simulink library "commchan"  (Simulink 5.0)
values from neighbouring files (symbols this model uses):
  b = []    [commblkvfdly.m]    (also in eyesampl.m = findobj(a, 'Name', get_param(gcbh,'Name')))
  params = []    [commblkeyescatdisc.m]
undefined symbols (not defined in the file or in its folder): j
libraries: dspsrcs2 x2, commsource x2, dspmlti2 x2, dsparch2 x1, dspelem2 x1, dspmtrx2 x1, commchan x1
settings Model: RequirementInfo=9  Creator=tdelve  LastModifiedBy=mmclerno

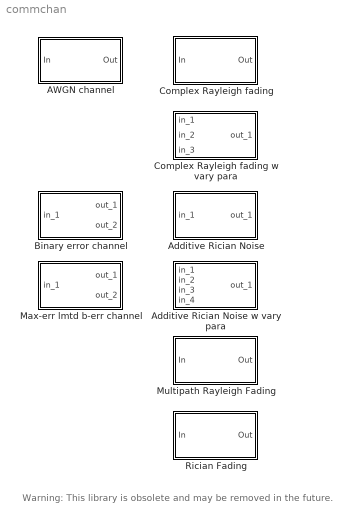
== system commchan ==
  note: Warning:  This library is obsolete and may
      | be removed in the future.
  AWGN channel : Subsystem  mask(AWGN Channel){seed=123456, noiseMode=Signal to noise ratio  (Es/No), EsNodB=10, SNRdB=10, Ps=1, Tsym=1, variance=1, FrameBased=off, nChans=1}
      mask prompts: seed "Initial seed:"; noiseMode "Mode:"; EsNodB "Es/No (dB):"; SNRdB "SNR (dB):"; Ps "Input signal power (Watts):"; Tsym "Symbol period (sec):"; FrameBased "Frame-based inputs"; nChans "Number of channels:"
      mask help:
      | Add white Gaussian noise to the input signal. The input and output signals can be real or complex. This block supports multi channel input and output signals as well as frame-based processing.
      |
      | When using either of the variance modes with complex inputs, the variance values are equally divided among the real and imaginary components of the input signal.
      mask init:
      | [mode,s]=commblkawgnchan(gcb,'init');
      mask StyleString: edit,popup(Signal to noise ratio  (Es/No)|Signal to noise ratio  (SNR)|Variance from mask|Variance from port),edit,edit,edit,edit,edit,checkbox,edit
      mask CallbackString: |commblkawgnchan(gcb,'Mode');||||||commblkawgnchan(gcb,'FrameBased');|
      mask Display:
      | plot(-10,-10,110, 110,[05 15 10 10 05 10 18 14 13 7.5 13 41 44 47 50 53 57
      | 59 100-[13 7.5 13 14 18 10 5 10 10 15 5]],[70 70 70 85 92 85 79 82 90 88.5
      | 90 90 87 93 87 93 87 90 90 88.5 90 82 79 85 92 85 70 70 70]);
      | disp('AWGN');
      | port_label('input',s.i1,s.i1s);
      | port_label('input',s.i2,s.i2s);
      | port_label('output',s.o1,s.o1s);
  Additive Rician Noise : Subsystem  mask(Rician noise channel, fixed parameter){m1=.1, m2=.3, d=.1, s=1234}
      mask prompts: m1 "In-phase mean:"; m2 "Quadrature mean:"; d "Variance:"; s "Seed:"
      mask help: Additive Rician noise channel for baseband signal simulation. Input and output signals are complex.
      mask init:
      | rand('state',s(1));
      | SeedVec = floor(1e5*rand(2,1));
      mask Help: This block adds Rician noise to the input signal. The input and output of this block are complex signals. Rician noise is composed of two independant Gaussian noise elements. The two Gaussian components have the same variance. Their mean values are in-phase mean and quadrature mean respectively.
      mask Display:
      | plot(0,0,100,100,[05 15 10 10 05 10 18 14 13 7.5 13 41 44 47 50 53 57 59 100-[13 7.5 13 14 18 10 5 10 10 15 5]],[70 70 70 85 92 85 79 82 90 88.5 90 90 87 93 87 93 87 90 90 88.5 90 82 79 85 92 85 70 70 70]);
      | disp('Complex\nRician Noise')
  Additive Rician Noise w vary para : Subsystem  mask(Rician noise channel, vary parameter){s=[13579,  24680]}
      mask prompts: s "Seeds:"
      mask help: Add Rician noise to complex signal (1st port) with the varying in-phase mean (2nd port), quadrature mean (3rd port), and variance (4th port).
      mask init:
      | rand('state',s(1));
      | SeedVec = floor(1e5*rand(2,1));
      mask Help: This block adds Rician noise to the transmitted signal. The 1st port input and output of this block are complex data. The Rician noise is composed of two independant Gaussian noise elements. The mean value of the two Gaussian components are input from 2nd and 3rd inports respectively. Their variance are the same which is input from the 4th inport.
      mask Display:
      | plot(0,0,100,100,[05 15 10 10 05 10 18 14 13 7.5 13 41 44 47 50 53 57 59 100-[13 7.5 13 14 18 10 5 10 10 15 5]],[70 70 70 85 92 85 79 82 90 88.5 90 90 87 93 87 93 87 90 90 88.5 90 82 79 85 92 85 70 70 70]);
      | disp('Complex\nRician Noise')
  Binary error channel : Subsystem  mask(Binary Error Channel){P=0.05, M=15, s=12345, Ts=1}
      mask prompts: P "Error probability:"; M "Input vector length:"; s "Seed"; Ts "Sample time (s):"
      mask help: Add binary errors to the input signal. The error probability can be a scalar or a vector with the same length as the input vector length.
      mask init:
      | if length(P)~=M,P=ones(1,M)*P(1);end;
      | seed = s(1)+cumsum(ones(1,M));
      mask Help: This block adds binary errors to transmitted binary signals. The error probability is given in the parameter setting. The first output port outputs the transmitting signal (after adding noise). The second port outputs the errors signal added to the transmitting signal.
      mask Display:
      | plot(0,0,100,100,[05 15 10 10 05 10 18 14 13 7.5 13 41 44 47 50 53 57 59 100-[13 7.5 13 14 18 10 5 10 10 15 5]],[70 70 70 85 92 85 79 82 90 88.5 90 90 87 93 87 93 87 90 90 88.5 90 82 79 85 92 85 70 70 70]);
      | disp('B-error')
  Complex Rayleigh fading : Subsystem  mask(Rayleigh fading channel, fixed parameter){a=1, Ph=0}
      mask prompts: a "Rayleigh fading envelope:"; Ph "Phase shift of the channel (rad):"
      mask help: Rayleigh fading channel with fixed fading envelope and phase shift.
      mask Help: This block applies the fading and phase shifting to the transmitting signal. In general, the fading envelope should be no larger than one. The input and the output of this block are both complex signals.
      mask Display:
      | plot(0,0,100,100,[05 15 10 10 05 10 18 14 13 7.5 13 41 44 47 50 53 57 59 100-[13 7.5 13 14 18 10 5 10 10 15 5]],[70 70 70 85 92 85 79 82 90 88.5 90 90 87 93 87 93 87 90 90 88.5 90 82 79 85 92 85 70 70 70]);
      | disp('Complex\nRayl Fading')
  Complex Rayleigh fading w vary para : Subsystem
      mask Type: Rayleigh fading channel, vary parameter
      mask Description: The fading envelope and the phase shift of the channel changes with the 2nd and 3rd input port values.
      mask Help: This block applies Rayleigh fading to the transmitting signals. The fading envelope and the phase of the channel are provided in the 2nd and the 3rd input port. The 1st input port and the output of this block are complex signals.
      mask Display:
      | plot(0,0,100,100,[05 15 10 10 05 10 18 14 13 7.5 13 41 44 47 50 53 57 59 100-[13 7.5 13 14 18 10 5 10 10 15 5]],[70 70 70 85 92 85 79 82 90 88.5 90 90 87 93 87 93 87 90 90 88.5 90 82 79 85 92 85 70 70 70]);
      | disp('Complex\nRayl Fading')
  Max-err lmtd b-err channel : Subsystem  mask(Limited binary error channel){leng=7, prob=1/2, seed=12345, Ts=}
      mask prompts: leng "Vector length(can't be changed during simulation):"; prob "Probability of one err, two errs, three errs...:"; Ts "Sample time (s):"
      mask help: Add binary errors with specified error number probability.
      mask Help: This block adds binary errors to the input signal. The maximum number of errors added to the signal is the same as the length of the vector probability. The value of ith element of the probability is the probability of i number of errors in the vector. The 1st outport is the signal with added noise. The 2nd outport is the added noise.
      mask Display:
      | plot(0,0,100,100,[05 15 10 10 05 10 18 14 13 7.5 13 41 44 47 50 53 57 59 100-[13 7.5 13 14 18 10 5 10 10 15 5]],[70 70 70 85 92 85 79 82 90 88.5 90 90 87 93 87 93 87 90 90 88.5 90 82 79 85 92 85 70 70 70]);
      | disp('Lmtd b-err')
  Multipath Rayleigh Fading : Subsystem  mask(Multipath Rayleigh Fading){Fd=40, simTs=1e-6, delayVec=[0 2e-6], gainVecdB=[0 -3], normGain=on, Seed=1234}
      mask prompts: Fd "Doppler frequency (Hz):"; simTs "Sample time (sec):"; delayVec "Delay vector (sec):"; gainVecdB "Gain vector (dB):"; normGain "Normalize gain vector to 0 dB overall gain"; Seed "Initial seed:"
      mask help:
      | Multipath Rayleigh fading channel for complex baseband signals.
      |
      | Multiplies the input signal with samples of a Rayleigh distributed complex random process. The spectrum of the Rayleigh process is given by the Jakes PSD, where the Doppler frequency parameter determines the maximum Doppler frequency.
      |
      | The number of paths equals the length of either the 'Delay vector' or 'Gain vector' parameters.
      mask init:
      | commblkrayleighchan(gcb);
      mask Help: web(commbhelp);
      mask Display:
      | plot(0,0,100,100,[05 15 10 10 05 10 18 14 13 7.5 13 41 44 47 50 53 57 59 100-[13 7.5 13 14 18 10 5 10 10 15 5]],[70 70 70 85 92 85 79 82 90 88.5 90 90 87 93 87 93 87 90 90 88.5 90 82 79 85 92 85 70 70 70]);
      | disp('Multipath\nRayleigh Fading')
  Rician Fading : Subsystem  mask(Rician Fading){K=1, Fd=40, simTs=1e-6, delayVec=0, gainVecdB=0, Seed=1234}
      mask prompts: K "K-factor:"; Fd "Doppler frequency (Hz):"; simTs "Sample time (sec):"; delayVec "Delay (sec):"; gainVecdB "Gain (dB):"; Seed "Initial seed:"
      mask help:
      | Rician fading channel for complex baseband signals.
      |
      | Multiplies the input signal with samples of a Rician distributed complex random process. The K-factor parameter specifies the linear ratio of power in the direct path to the diffuse power.  The spectrum of the Rician process is given by the Jakes PSD, where the Doppler frequency parameter determines the maximum Doppler frequency.
      mask init:
      | commblkricianchan(gcb);
      mask Help: web(commbhelp);
      mask Display:
      | plot(0,0,100,100,[05 15 10 10 05 10 18 14 13 7.5 13 41 44 47 50 53 57 59 100-[13 7.5 13 14 18 10 5 10 10 15 5]],[70 70 70 85 92 85 79 82 90 88.5 90 90 87 93 87 93 87 90 90 88.5 90 82 79 85 92 85 70 70 70]);
      | disp('Rician\nFading')

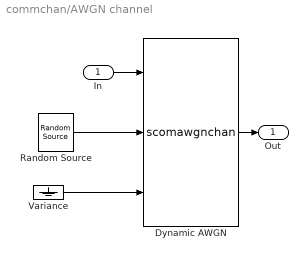
== system commchan/AWGN channel ==
  In : Inport
  Dynamic AWGN : S-Function  FunctionName=scomawgnchan  Parameters=noiseMode,EsNodB,SNRdB,Ps,Tsym,variance,FrameBased,nChans
  Random Source : dspsrcs2/Random Source  SrcType=Gaussian  Min=0  Max=1  Mean=0  Var=1  Seed=seed  SampMode=Discrete  Inherit=on  SampTime=1  SampFrame=1  OutComplex=Real
  Variance : Ground
  Out : Outport
  wires:
  Random Source/1 -> Dynamic AWGN/2
  In/1 -> Dynamic AWGN/1
  Dynamic AWGN/1 -> Out/1
  Variance/1 -> Dynamic AWGN/3

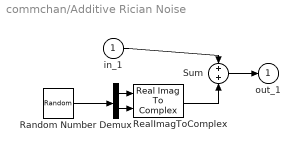
== system commchan/Additive Rician Noise ==
  in_1 : Inport
  Demux : Demux  Outputs=2
  Random Number : RandomNumber  Mean=[m1 m2]  Variance=[d d]  Seed=SeedVec
  RealImagToComplex : RealImagToComplex
  Sum : Sum  SaturateOnIntegerOverflow=on  InputSameDT=on
  out_1 : Outport  InitialOutput=0
  wires:
  Sum/1 -> out_1/1
  in_1/1 -> Sum/1
  RealImagToComplex/1 -> Sum/2
  Demux/1 -> RealImagToComplex/1
  Demux/2 -> RealImagToComplex/2
  Random Number/1 -> Demux/1

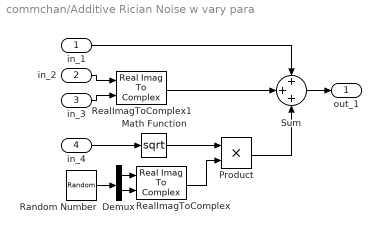
== system commchan/Additive Rician Noise w vary para ==
  in_1 : Inport
  in_2 : Inport  Port=2
  in_3 : Inport  Port=3
  in_4 : Inport  Port=4
  Demux : Demux  Outputs=2
  Math Function : Math  Operator=sqrt
  Product : Product  SaturateOnIntegerOverflow=on  InputSameDT=on
  Random Number : RandomNumber  Seed=SeedVec
  RealImagToComplex : RealImagToComplex
  RealImagToComplex1 : RealImagToComplex
  Sum : Sum  Inputs=+++  SaturateOnIntegerOverflow=on  InputSameDT=on
  out_1 : Outport  InitialOutput=0
  wires:
  in_2/1 -> RealImagToComplex1/1
  in_3/1 -> RealImagToComplex1/2
  RealImagToComplex/1 -> Product/2
  Product/1 -> Sum/3
  RealImagToComplex1/1 -> Sum/2
  in_1/1 -> Sum/1
  Sum/1 -> out_1/1
  Demux/1 -> RealImagToComplex/1
  Demux/2 -> RealImagToComplex/2
  Random Number/1 -> Demux/1
  in_4/1 -> Math Function/1
  Math Function/1 -> Product/1

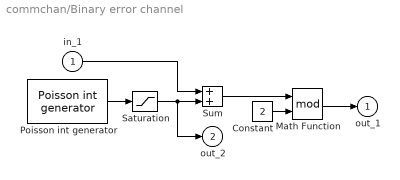
== system commchan/Binary error channel ==
  in_1 : Inport
  Constant : Constant  Value=2
  Math Function : Math  Operator=mod
  Poisson int generator : commsource/Poisson int generator  lambda=P  seed=seed  Ts=Ts
  Saturation : Saturate  UpperLimit=1  LowerLimit=0
  Sum : Sum  SaturateOnIntegerOverflow=on  InputSameDT=on
  out_1 : Outport  InitialOutput=0
  out_2 : Outport  Port=2  InitialOutput=0
  wires:
  Saturation/1 -> Sum/2, out_2/1
  Poisson int generator/1 -> Saturation/1
  in_1/1 -> Sum/1
  Sum/1 -> Math Function/1
  Constant/1 -> Math Function/2
  Math Function/1 -> out_1/1

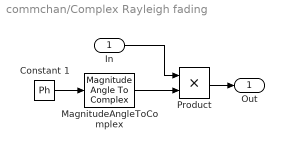
== system commchan/Complex Rayleigh fading ==
  In : Inport
  Constant 1 : Constant  Value=Ph
  MagnitudeAngleToComplex : MagnitudeAngleToComplex  Input=Angle  ConstantPart=a
  Product : Product  SaturateOnIntegerOverflow=on  InputSameDT=on
  Out : Outport  InitialOutput=0
  wires:
  Constant 1/1 -> MagnitudeAngleToComplex/1
  MagnitudeAngleToComplex/1 -> Product/2
  In/1 -> Product/1
  Product/1 -> Out/1

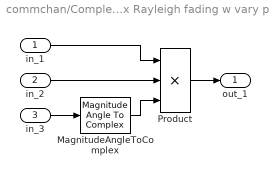
== system commchan/Complex Rayleigh fading w vary para ==
  in_1 : Inport
  in_2 : Inport  Port=2
  in_3 : Inport  Port=3
  MagnitudeAngleToComplex : MagnitudeAngleToComplex  Input=Angle  ConstantPart=1
  Product : Product  Inputs=3  SaturateOnIntegerOverflow=on  InputSameDT=on
  out_1 : Outport  InitialOutput=0
  wires:
  Product/1 -> out_1/1
  in_2/1 -> Product/2
  in_1/1 -> Product/1
  MagnitudeAngleToComplex/1 -> Product/3
  in_3/1 -> MagnitudeAngleToComplex/1

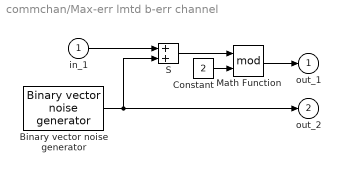
== system commchan/Max-err lmtd b-err channel ==
  in_1 : Inport
  Binary vector noise generator : commsource/Binary vector noise generator  n=leng  prob=prob  seed=seed  Ts=Ts
  Constant : Constant  Value=2
  Math Function : Math  Operator=mod
  S : Sum  SaturateOnIntegerOverflow=on  InputSameDT=on
  out_1 : Outport  InitialOutput=0
  out_2 : Outport  Port=2  InitialOutput=0
  wires:
  S/1 -> Math Function/1
  in_1/1 -> S/1
  Binary vector noise generator/1 -> S/2, out_2/1
  Constant/1 -> Math Function/2
  Math Function/1 -> out_1/1

== system commchan/Multipath Rayleigh Fading ==
  In : Inport
  Multipath Fading Channel : Subsystem  mask(Multipath Fading){Fd=Fd, LOSFd=0, K=0, simTs=simTs, delayVec=delayVec, gainVecdB=gainVecdB, normGain=on, Seed=Seed}
      mask prompts: Fd "Doppler frequency (Hz):"; LOSFd "Line-of-sight Doppler frequency (Hz):"; K "K-factor:"; simTs "Sample time (sec):"; delayVec "Delay vector (sec):"; gainVecdB "Gain vector (dB):"; normGain "Normalize gain vector to 0 dB overall gain"; Seed "Initial seed:"
      mask help:
      | Multipath fading channel for complex baseband signals.
      |
      | Multiplies the input signal with samples of a complex random process. The spectrum of the random process is given by the Jakes PSD, where the Doppler frequency parameter determines the maximum Doppler frequency. The K-factor parameter specifies the linear ratio of power in the direct path to the diffuse power.
      |
      | The number of paths equals the length of either the 'Delay vector' or 'Gain vector' parameters.
      mask init:
      | [ecode,emsg,params] = commblkfadingchan(gcb,Fd,LOSFd,K,simTs,delayVec,gainVecdB,normGain,Seed);
      | if(ecode==1)
      |     error(emsg);
      | elseif(ecode==2)
      |     warning(emsg);
      | end;
      mask Display:
      | plot(0,0,100,100,[05 15 10 10 05 10 18 14 13 7.5 13 41 44 47 50 53 57 59 100-[13 7.5 13 14 18 10 5 10 10 15 5]],[70 70 70 85 92 85 79 82 90 88.5 90 90 87 93 87 93 87 90 90 88.5 90 82 79 85 92 85 70 70 70]);
      | disp('Multipath\nFading')
  Out : Outport
  wires:
  In/1 -> Multipath Fading Channel/1(In)
  Multipath Fading Channel/1(Out) -> Out/1

== system commchan/Rician Fading ==
  In : Inport
  Multipath Fading Channel : commchan/Multipath Rayleigh Fading/Multipath Fading Channel  Fd=Fd  LOSFd=0  K=K  simTs=simTs  delayVec=delayVec  gainVecdB=gainVecdB  normGain=off  Seed=Seed
  Out : Outport
  wires:
  In/1 -> Multipath Fading Channel/1
  Multipath Fading Channel/1 -> Out/1

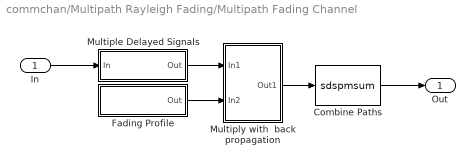
== system commchan/Multipath Rayleigh Fading/Multipath Fading Channel ==
  In : Inport
  Combine Paths : S-Function  FunctionName=sdspmsum  Parameters=Cols,Dim  mask(Matrix Sum){Dim=Rows, Cols=params.nPaths}
      mask prompts: Dim "Sum along:"; Cols "Number of columns in input:"
      mask help: Sum of matrix elements along the row or column dimension.
      mask init:
      | if (Dim==1), str='Row\nSum';
      | else str='Column\nSum';
      | end
      mask Help: web(dspbhelp);
      mask StyleString: popup(Rows|Columns),edit
      mask Display: disp(str);
  Fading Profile : Subsystem
      mask Display: disp('Fading\nProfile')
  Multiple Delayed Signals : Subsystem  mask(Multiple Delayed Signals){delayVector=params.sampleDelayVec, Ts=simTs}
      mask prompts: delayVector "Path delay vector:"; Ts "Sample time (sec):"
      mask init:
      | nPaths = length(delayVector);
      | maxDelay = ceil(max(delayVector))+1;
      mask Display: disp('Multiple\ndelayed signals');
  Multiply with  back propagation : Subsystem  mask(Multiply with back propagation){propTarget=Input 2, Ts=simTs, numChan=params.nPaths}
      mask prompts: propTarget "Propagation target:"; Ts "Sample time:"; numChan "Number of channels:"
      mask help:
      | Perform multiplication of the two input signals.
      |
      | The width and complexity of the output and the port not targeted for propagation must be identical. The width and complexity of the port targeted for propagation is set to that of the other input.
      |
      | The block sample time is the product of the number of samples per frame and the sample time parameter.
      mask StyleString: popup(Input 1|Input 2),edit,edit
      mask Display: disp('Multiply\nwith prop');
  Out : Outport
  wires:
  Multiple Delayed Signals/1(Out) -> Multiply with  back propagation/1(In1)
  Fading Profile/1(Out) -> Multiply with  back propagation/2(In2)
  In/1 -> Multiple Delayed Signals/1(In)
  Multiply with  back propagation/1(Out1) -> Combine Paths/1
  Combine Paths/1 -> Out/1

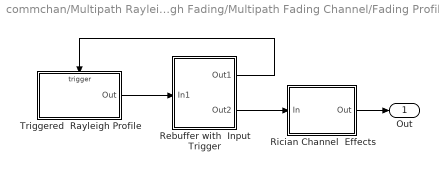
== system commchan/Multipath Rayleigh Fading/Multipath Fading Channel/Fading Profile ==
  Rebuffer with  Input Trigger : Subsystem  mask(Rebuffer with Input Trigger){startSample=params.startDelay, numChan=params.nPaths, inputWidthMode=Based on output width, inputWidth=params.intFactor, inputWidthMin=params.intFactor, inputWidthStep=params.intFactor, inputWidthMax=params.maxPathWidth}
      mask prompts: startSample "Start delay:"; numChan "Number of channels:"; inputWidthMode "Input width mode:"; inputWidth "Input width (per channel):"; inputWidthMin "Minimum input width (per channel):"; inputWidthStep "Input width step size (per channel):"; inputWidthMax "Maximum input width (per channel):"
      mask help: This block inherits the input and output port widths and complexity and the output sample time. The input must be from a function call subsystem. The block generates a function call trigger on port 1 when ever data is required. and outputs the buffered input data on port 2.
      mask init:
      | s = commblktriggeredbuffer(gcb,'init',{});
      mask StyleString: edit,edit,popup(Inherit|Specify|Based on output width),edit,edit,edit,edit
      mask CallbackString: ||commblktriggeredbuffer(gcb,'InputWidthMode');||||
      mask Display:
      | disp('Rebuffer\nwith trigger');
      | port_label('input',s.i1,s.i1s);
      | port_label('output',s.o1,s.o1s);
      | port_label('output',s.o2,s.o2s);
  Rician Channel  Effects : Subsystem  mask(Ricean Channel Effects){Doppler=params.LOSFd, K=params.K, opPower=params.gainVecLin, Ts=simTs, numChan=params.nPaths}
      mask prompts: Doppler "Line-of-sight Doppler frequency (Hz):"; K "K-factor"; opPower "Required output power (Watts):"; Ts "Sample time (s):"; numChan "Number of channels:"
      mask help: Add a complex phasor to the unity variance complex input to produce Rician channel effects. The Doppler frequency parameter determines frequency of the complex phasor.
      mask Display: disp('Rician\nChannel')
  Triggered  Rayleigh Profile : Subsystem  TreatAsAtomicUnit=on
  Out : Outport
  wires:
  Rebuffer with  Input Trigger/1(Out1) -> Triggered  Rayleigh Profile/Trigger
  Triggered  Rayleigh Profile/1(Out) -> Rebuffer with  Input Trigger/1(In1)
  Rebuffer with  Input Trigger/2(Out2) -> Rician Channel  Effects/1(In)
  Rician Channel  Effects/1(Out) -> Out/1

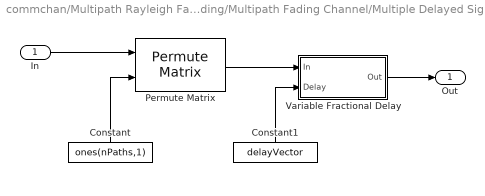
== system commchan/Multipath Rayleigh Fading/Multipath Fading Channel/Multiple Delayed Signals ==
  In : Inport
  Constant : Constant  Orientation=up  Value=ones(nPaths,1)
  Constant1 : Constant  Orientation=up  Value=delayVector
  Permute Matrix : dspmtrx2/Permute Matrix  mode=Columns  errmode=Clip Index  cols=1
  Variable Fractional Delay : Subsystem  mask(Variable Fractional Delay){mode=FIR Interpolation, dmax=maxDelay, L=6, R=10, alpha=1, ic=0, frame=on, numChans=nPaths, delayMode=on}
      mask prompts: dmax "Maximum delay in samples:"; L "Interpolation filter half-length:"; R "Interpolation points per input sample:"; alpha "Normalized input bandwidth (0 to 1):"; ic "Initial Conditions:"; frame "Frame-Based Inputs"; numChans "Number of Channels:"; delayMode "Delay input is "delay per channel""
      mask help: Delay discrete-time input by a time-varying fractional number of sample periods, as specified by the "delay" input. The delay may be applied on an element-by-element basis or channel-by-channel. Delay must be a real vector signal with one delay value per frame element or one delay value per channel when in channel-by-channel mode. The FIR filter is designed using "intfilt" from the Signal Processing Toolbox.
      mask init:
      | [b,str] = commblkvfdly(mode,R,L,alpha);
      | if strcmp(frame,'off'), numChans=-1; end
      mask StyleString: popup(Linear Interpolation|FIR Interpolation),edit,edit,edit,edit,edit,checkbox,edit,checkbox
      mask CallbackString: commblkvfdly||||||commblkvfdly||
      mask Display:
      | text(0.5,0.4,'z','horiz','right')
      | text(0.5,0.6,'-f','horiz','left')
  Out : Outport
  wires:
  Constant/1 -> Permute Matrix/2
  Permute Matrix/1 -> Variable Fractional Delay/1(In)
  Constant1/1 -> Variable Fractional Delay/2(Delay)
  Variable Fractional Delay/1(Out) -> Out/1
  In/1 -> Permute Matrix/1

== system commchan/Multipath Rayleigh Fading/Multipath Fading Channel/Multiply with  back propagation ==
  In1 : Inport
  In2 : Inport  Port=2
  S-Function : S-Function  FunctionName=scommultwithprop  Parameters=propTarget, Ts, numChan
  Out1 : Outport
  wires:
  S-Function/1 -> Out1/1
  In1/1 -> S-Function/1
  In2/1 -> S-Function/2

== system commchan/Multipath Rayleigh Fading/Multipath Fading Channel/Fading Profile/Rebuffer with  Input Trigger ==
  In1 : Inport
  S-Function : S-Function  FunctionName=scomtrigbuff  Parameters=startSample, numChan, inputWidthMode, inputWidth, inputWidthMin, inputWidthStep, inputWidthMax
  Out1 : Outport
  Out2 : Outport  Port=2
  wires:
  In1/1 -> S-Function/1
  S-Function/2 -> Out2/1
  S-Function/1 -> Out1/1

== system commchan/Multipath Rayleigh Fading/Multipath Fading Channel/Fading Profile/Rician Channel  Effects ==
  In : Inport
  S-Function : S-Function  FunctionName=scomricianlos  Parameters=Doppler,K,opPower,Ts,numChan
  Out : Outport
  wires:
  S-Function/1 -> Out/1
  In/1 -> S-Function/1

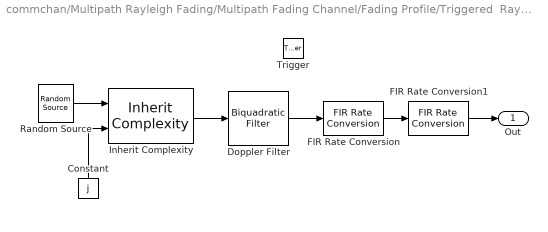
== system commchan/Multipath Rayleigh Fading/Multipath Fading Channel/Fading Profile/Triggered  Rayleigh Profile ==
  Trigger : TriggerPort  TriggerType=function-call
  Constant : Constant  Orientation=up  Value=j
  Doppler Filter : dsparch2/Biquadratic Filter  sos=params.dopplerSos  ic=0  frame=on  nchans=params.nPaths
  FIR Rate Conversion : dspmlti2/FIR Rate Conversion  L=params.interp1  h=params.interp1Num  M=1  numChans=params.nPaths
  FIR Rate Conversion1 : dspmlti2/FIR Rate Conversion  L=params.interp2  h=params.interp2Num  M=1  numChans=params.nPaths
  Inherit Complexity : dspelem2/Inherit Complexity
  Random Source : dspsrcs2/Random Source  SrcType=Gaussian  Min=0  Max=1  Mean=zeros(params.nPaths,1)  Var=ones(params.nPaths,1)  Seed=params.Seed  SampMode=Discrete  Inherit=on  SampTime=1  SampFrame=1  OutComplex=Real
  Out : Outport
  wires:
  Random Source/1 -> Inherit Complexity/1
  Constant/1 -> Inherit Complexity/2
  Inherit Complexity/1 -> Doppler Filter/1
  FIR Rate Conversion/1 -> FIR Rate Conversion1/1
  Doppler Filter/1 -> FIR Rate Conversion/1
  FIR Rate Conversion1/1 -> Out/1

== system commchan/Multipath Rayleigh Fading/Multipath Fading Channel/Multiple Delayed Signals/Variable Fractional Delay ==
  In : Inport
  Delay : Inport  Port=2
  S-Function : S-Function  FunctionName=scomvfdly  Parameters=dmax,b,ic,numChans,delayMode
  Out : Outport  InitialOutput=0
  wires:
  S-Function/1 -> Out/1
  Delay/1 -> S-Function/2
  In/1 -> S-Function/1
